simulink model "bus_replicate_blk"  (R2019a)
settings: Solver=VariableStepAuto  StartTime=0.0  StopTime=10.0  RelTol=1e-3
libraries: xbsIndex_r4 x4
settings Model: Creator=Ross Donnachie  LastModifiedBy=Ross Donnachie

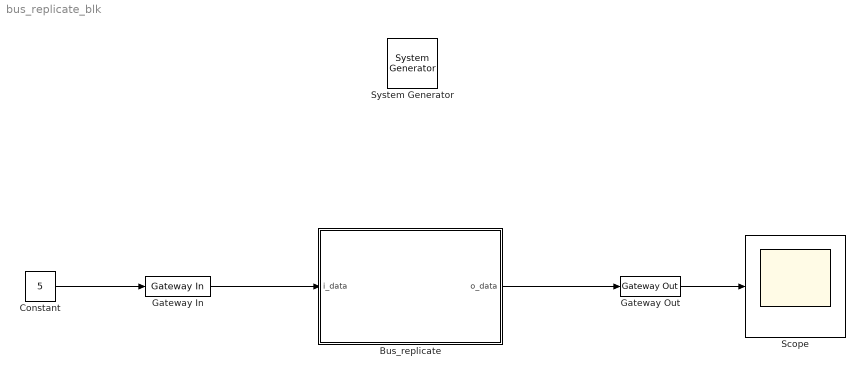
== system bus_replicate_blk ==
  " System Generator" : xbsIndex_r4/ System Generator  Tag=genX  xilinxfamily=kintex7  part=xc7k325t  speed=-3  package=fbg676  synthesis_tool=Vivado  clock_wrapper=Clock Enables  directory=./netlist  proj_type=Vivado  Synth_file=Vivado Synthesis Defaults  Impl_file=Vivado Implementation Defaults  testbench=off  simulink_period=1  sysclk_period=10  dcm_input_clock_period=10  incr_netlist=off  trim_vbits=Everywhere in SubSystem  dbl_ovrd=According to Block Masks  core_generation=According to Block Masks  run_coregen=off  deprecated_control=off  eval_field=0  block_type=sysgen
  Bus_replicate : Subsystem  mask{replication_factor=2, delay=0, misc_enabled=off}
      mask prompts: replication_factor "Replication Factor"; delay "Latency"; misc_enabled "Misc Support"
      mask DialogControl DescTextVar Prompt: Output bus formed with the input repeated in each element.
  Constant : Constant  Value=5
  Gateway In : xbsIndex_r4/Gateway In  gui_display_data_type=Fixed-point  arith_type="Signed  (2's comp)"  n_bits=5  bin_pt=0  preci_type=Single  exp_width=8  frac_width=24  rows=1  columns=1  quantization="Round  (unbiased: +/- Inf)"  overflow=Saturate  period=1  UseAsADC=off  ADCChannel='1'  interface=None  automatic_assignment=on  address_offset=hex2dec('00')  intf_name=''  intf_description=''  default_value=0  timing_constraint=None  locs_specified=off  LOCs={}  io_standard={}  inherit_from_input=off  hdl_port=on  dbl_ovrd=off  block_type=gatewayin
  Gateway Out : xbsIndex_r4/Gateway Out  inherit_from_input=off  hdl_port=on  rows=1  columns=1  UseAsDAC=off  DACChannel='1'  interface=None  automatic_assignment=on  address_offset=hex2dec('00')  intf_name=''  intf_description=''  timing_constraint=None  locs_specified=off  LOCs={}  io_standard={}  block_type=gatewayout
  Scope : Scope
  wires:
  Constant/1 -> Gateway In/1
  Gateway In/1 -> Bus_replicate/1(i_data)
  Bus_replicate/1(o_data) -> Gateway Out/1
  Gateway Out/1 -> Scope/1

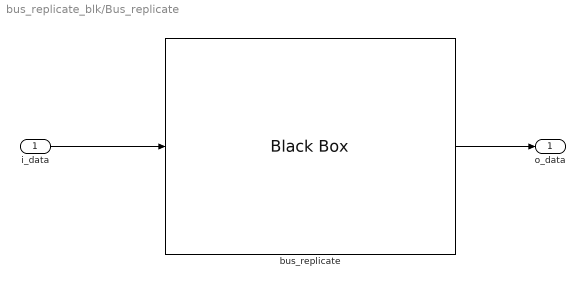
== system bus_replicate_blk/Bus_replicate ==
  i_data : Inport
  bus_replicate : xbsIndex_r4/Black Box  init_code=bus_replicate_config  sim_method=ISE Simulator  verbose=off  block_type=blackbox2
  o_data : Outport
  wires:
  i_data/1 -> bus_replicate/1
  bus_replicate/1 -> o_data/1
